simulink model "PubIfDecisionVSM_SetSpd"  (R2020b)
settings: Solver=FixedStepAuto  StartTime=0.0  StopTime=Inf  RelTol=1e-3
PostLoadFcn:
  | if any(exist('dsrtsu_mdlpostloadfcn', 'file') ~= 0), dsrtsu_mdlpostloadfcn('Execute', bdroot); end
InitFcn:
  | , if any(exist('dsmpb_private', 'file') ~= 0), dsmpb_private('dsmpb_mdlclblib', 'Init', bdroot); end,
PreSaveFcn:
  | , if any(exist('dsmpb_private', 'file') ~= 0), dsmpb_private('dsmpb_mdlclblib', 'PreSave', bdroot); end,
CloseFcn:
  | , if any(exist('dsmpb_private', 'file') ~= 0), dsmpb_private('dsmpb_mdlclblib', 'Close', bdroot); end,
settings Model: DataDictionary=HWA_DDs.sldd  RTICANMMDATA=struct('GeneralSetupData',struct('modelroot','D:\ADAS_Store\Adas\VSM\SetSpd_TimeGap','generalsettings',struct('filesettings',struct('destfolder',struct('Name','RTICANMM_FILES','Check',1),'buildfolder',struct('Name','.','Check',1),'AbsDestfolder',struct('Name','D:\ADAS_Store\Adas\VSM\SetSpd_TimeGap\RTICANMM_FILES'),'AbsBuildfolder',struct('Name','D:\ADAS_Store\Adas\VSM\SetSpd_TimeGap'))),'options',struct('addpaths',1,'rmpaths',1,'addtrcexclusion',false,'cannavigator',struct('checkmonitoring',0),'show_usrtrc',0,'use_usrtrc',0),'advanced',struct('options',ones(1,100)),'MPSetup',{{}},'RTI',struct('Type','DSRT','Ver','4.2','Date','02-Nov-2019'),'modelname','PubIfDecisionVSM_SetSpd','block','PubIfDecisionVSM_SetSpd'))  DSRTSU_INTERNAL_RTIFPGA=150  Creator=GW00180895  LastModifiedBy=GW00166368
settings OptimizationCC: BlockReduction=off  ConditionallyExecuteInputs=off  OptimizeBlockIOStorage=off  BufferReuse=off  GlobalBufferReuse=off  ExpressionFolding=off  LocalBlockOutputs=off  OptimizeDataStoreBuffers=off  BusAssignmentInplaceUpdate=off
settings DebuggingCC: TasksWithSamePriorityMsg=none
settings HardwareCC: ProdBitPerPointer=32  ProdBitPerSizeT=32  ProdBitPerPtrDiffT=32  ProdLargestAtomicInteger=Integer  ProdWordSize=32  ProdHWDeviceType=Custom Processor->Custom
settings ModelReferenceCC: UpdateModelReferenceTargets=IfOutOfDate  EnableParallelModelReferenceBuilds=on  ModelReferenceNumInstancesAllowed=Single
settings SFSimCC: MATLABDynamicMemAlloc=off
settings RTWCC: Description=dSPACE Run-Time Target (for VEOS on Windows and ConfigurationDesk)  SystemTargetFile=dsrt.tlc  GenCodeOnly=on  MakeCommand=make_dsrt  TemplateMakefile=dsrt_default_tmf  RTWVerbose=off
settings CodeAppCC: MaxIdLength=128
settings STFCustomTargetCC: TargetLangStandard=C99 (ISO)  ParMdlRefBuildCompliant=on  ConcurrentExecutionCompliant=off  CPPClassGenCompliant=off  GRTInterface=off  SystemTargetFile=dsrt.tlc
settings GRTTargetCC: CompOptLevelCompliant=off  ConcurrentExecutionCompliant=off  CombineOutputUpdateFcns=off  MatFileLogging=off  CPPClassGenCompliant=off  UseToolchainInfoCompliant=off

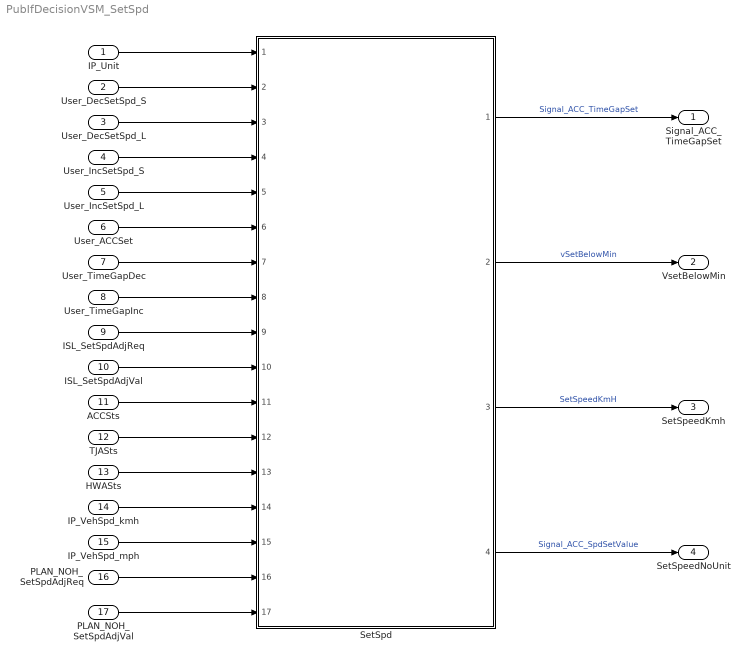
== system PubIfDecisionVSM_SetSpd ==
  IP_Unit : Inport  OutDataTypeStr=boolean
  User_DecSetSpd_S : Inport  Port=2  OutDataTypeStr=boolean
  User_DecSetSpd_L : Inport  Port=3  OutDataTypeStr=boolean
  User_IncSetSpd_S : Inport  Port=4  OutDataTypeStr=boolean
  User_IncSetSpd_L : Inport  Port=5  OutDataTypeStr=boolean
  User_ACCSet : Inport  Port=6  OutDataTypeStr=boolean
  User_TimeGapDec : Inport  Port=7  OutDataTypeStr=boolean
  User_TimeGapInc : Inport  Port=8  OutDataTypeStr=boolean
  ISL_SetSpdAdjReq : Inport  Port=9  OutDataTypeStr=boolean
  ISL_SetSpdAdjVal : Inport  Port=10  OutDataTypeStr=uint8
  ACCSts : Inport  Port=11  OutDataTypeStr=Enum: ACC_STATE
  TJASts : Inport  Port=12  OutDataTypeStr=Enum: TJA_STATE
  HWASts : Inport  Port=13  OutDataTypeStr=Enum: HWA_STATE
  IP_VehSpd_kmh : Inport  Port=14  OutDataTypeStr=single
  IP_VehSpd_mph : Inport  Port=15  OutDataTypeStr=single
  PLAN_NOH_SetSpdAdjReq : Inport  Port=16  OutDataTypeStr=boolean
  PLAN_NOH_SetSpdAdjVal : Inport  Port=17  OutDataTypeStr=uint8
  SetSpd : Subsystem  ReferencedSubsystem=PvtSubSys_VSM_SetSpd
  Signal_ACC_TimeGapSet : Outport  OutDataTypeStr=uint8
  VsetBelowMin : Outport  Port=2  OutDataTypeStr=boolean
  SetSpeedKmh : Outport  Port=3  OutDataTypeStr=single
  SetSpeedNoUnit : Outport  Port=4  OutDataTypeStr=uint8
  wires:
  User_ACCSet/1 -> SetSpd/6
  User_IncSetSpd_L/1 -> SetSpd/5
  User_TimeGapDec/1 -> SetSpd/7
  User_IncSetSpd_S/1 -> SetSpd/4
  User_TimeGapInc/1 -> SetSpd/8
  User_DecSetSpd_L/1 -> SetSpd/3
  ISL_SetSpdAdjReq/1 -> SetSpd/9
  User_DecSetSpd_S/1 -> SetSpd/2
  ISL_SetSpdAdjVal/1 -> SetSpd/10
  IP_Unit/1 -> SetSpd/1
  ACCSts/1 -> SetSpd/11
  TJASts/1 -> SetSpd/12
  HWASts/1 -> SetSpd/13
  IP_VehSpd_kmh/1 -> SetSpd/14
  IP_VehSpd_mph/1 -> SetSpd/15
  SetSpd/2 -> VsetBelowMin/1  "vSetBelowMin"
  SetSpd/1 -> Signal_ACC_TimeGapSet/1  "Signal_ACC_TimeGapSet"
  SetSpd/3 -> SetSpeedKmh/1  "SetSpeedKmH"
  SetSpd/4 -> SetSpeedNoUnit/1  "Signal_ACC_SpdSetValue"
  PLAN_NOH_SetSpdAdjReq/1 -> SetSpd/16
  PLAN_NOH_SetSpdAdjVal/1 -> SetSpd/17
